simulink model "saturateModel_15b"  (R2015b)
settings: Solver=FixedStepAuto  SolverMode=SingleTasking  StartTime=0.0  StopTime=30.0  FixedStep=0.01  RelTol=1e-3
InitFcn:
  | init
StopFcn:
  | res_plot
values from neighbouring files (symbols this model uses):
  g = 9.8    [init.m]    (also in main.m)
  I_1 = 1.25    [init.m]
  I_2 = 1.25    [init.m]
  I_3 = 2.5    [init.m]
  k_1_phi = 5.5    [init.m]
  k_1_psi = 8.5    [init.m]
  k_1_theta = 5.5    [init.m]
  k_2_phi = 10    [init.m]
  k_2_psi = 20    [init.m]
  k_2_theta = 10    [init.m]
  K_4 = 0.012    [init.m]
  K_5 = 0.012    [init.m]
  K_6 = 0.012    [init.m]
  k_d_x = 2.5    [init.m]
  k_d_y = 2.5    [init.m]
  k_d_z = 4.5    [init.m]
  k_p_x = 1.8    [init.m]
  k_p_y = 1.8    [init.m]
  k_p_z = 5.5    [init.m]
  k_phi = 1    [init.m]
  k_psi = 1    [init.m]
  k_theta = 1    [init.m]
  l = 0.20    (= 0.2)    [init.m]
  m = 2    [init.m]    (also in main.m = 0.5)
  M_phi = 25    [init.m]
  M_psi = 25    [init.m]
  M_theta = 25    [init.m]
  state0 = [0;0;0;0;0;0;0;0;0;0;0;0]    [init.m]    (also in main.m = [0;0;0;0;0;0;0;0;0.1;0;0;0])
  state_des = [4;4;5;pi/4]    [init.m]
undefined symbols (not defined in the file or in its folder): c, kf
settings Model: Creator=KingBoy  LastModifiedBy=KingBoy
settings DataIOCC: LimitDataPoints=off
settings DebuggingCC: AllowSymbolicDim=on  SFUnexpectedBacktrackingDiag=error  SFNoUnconditionalDefaultTransitionDiag=error
settings ModelReferenceCC: PropagateSignalLabelsOutOfModel=on
settings GRTTargetCC: TargetLangStandard=C99 (ISO)
settings ConfigComp: CovMetricSettings=dwe  CovHtmlReporting=off  CovSaveCumulativeToWorkspaceVar=off  CovSaveSingleToWorkspaceVar=off  CovModelRefEnable=Off  CovExternalEMLEnable=on

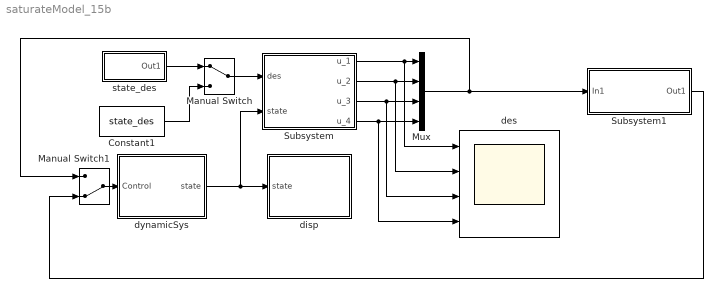
== system saturateModel_15b ==
  Constant1 : Constant  Value=state_des
  Manual Switch : ManualSwitch
  Manual Switch1 : ManualSwitch  CurrentSetting=0
  Mux : Mux
  Subsystem : Subsystem
  Subsystem1 : Subsystem
  des : Scope  NumInputPorts=4
  disp : Subsystem
  dynamicSys : Subsystem
  state_des : Subsystem
  wires:
  dynamicSys/1(state) -> disp/1(state), Subsystem/2(state)
  Constant1/1 -> Manual Switch/2
  Subsystem/1(u_1) -> des/1, Mux/1
  Subsystem/2(u_2) -> des/2, Mux/2
  Subsystem/3(u_3) -> des/3, Mux/3
  Subsystem/4(u_4) -> Mux/4, des/4
  Mux/1 -> Manual Switch1/1, Subsystem1/1(In1)
  state_des/1(Out1) -> Manual Switch/1
  Manual Switch/1 -> Subsystem/1(des)
  Subsystem1/1(Out1) -> Manual Switch1/2
  Manual Switch1/1 -> dynamicSys/1(Control)

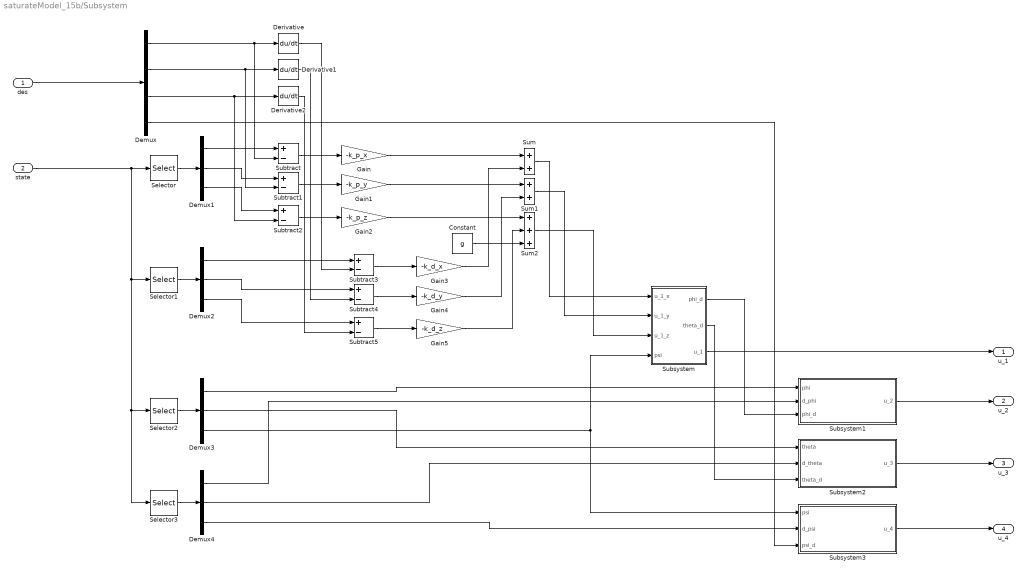
== system saturateModel_15b/Subsystem ==
  des : Inport
  state : Inport  Port=2
  Constant : Constant  Value=g
  Demux : Demux
  Demux{1..4} (4 alike) : Demux  Outputs=3
  Derivative : Derivative
  Derivative1 : Derivative
  Derivative2 : Derivative
  Gain : Gain  Gain=-k_p_x
  Gain1 : Gain  Gain=-k_p_y
  Gain2 : Gain  Gain=-k_p_z
  Gain3 : Gain  Gain=-k_d_x
  Gain4 : Gain  Gain=-k_d_y
  Gain5 : Gain  Gain=-k_d_z
  Selector : Selector  InputPortWidth=12  IndexOptions=Index vector (dialog)  Indices=[1:3]  OutputSizes=1
  Selector1 : Selector  InputPortWidth=12  IndexOptions=Index vector (dialog)  Indices=[4:6]  OutputSizes=1
  Selector2 : Selector  InputPortWidth=12  IndexOptions=Index vector (dialog)  Indices=[7:9]  OutputSizes=1
  Selector3 : Selector  InputPortWidth=12  IndexOptions=Index vector (dialog)  Indices=[10:12]  OutputSizes=1
  Subsystem : Subsystem
  Subsystem1 : Subsystem
  Subsystem2 : Subsystem
  Subsystem3 : Subsystem
  Subtract{,1..5} (6 alike) : Sum  Inputs=+-
  Sum : Sum
  Sum1 : Sum
  Sum2 : Sum  Inputs=+++
  u_1 : Outport
  u_2 : Outport  Port=2
  u_3 : Outport  Port=3
  u_4 : Outport  Port=4
  wires:
  state/1 -> Selector2/1, Selector3/1, Selector1/1, Selector/1
  des/1 -> Demux/1
  Demux/1 -> Subtract/2, Derivative/1
  Demux/2 -> Subtract1/2, Derivative1/1
  Demux/3 -> Subtract2/2, Derivative2/1
  Demux/4 -> Subsystem3/3(psi_d)
  Selector/1 -> Demux1/1
  Demux1/1 -> Subtract/1
  Demux1/2 -> Subtract1/1
  Demux1/3 -> Subtract2/1
  Selector1/1 -> Demux2/1
  Demux2/1 -> Subtract3/1
  Demux2/2 -> Subtract4/1
  Demux2/3 -> Subtract5/1
  Derivative/1 -> Subtract3/2
  Derivative1/1 -> Subtract4/2
  Derivative2/1 -> Subtract5/2
  Subtract/1 -> Gain/1
  Subtract2/1 -> Gain2/1
  Subtract1/1 -> Gain1/1
  Subtract3/1 -> Gain3/1
  Subtract4/1 -> Gain4/1
  Subtract5/1 -> Gain5/1
  Gain/1 -> Sum/1
  Gain1/1 -> Sum1/1
  Gain2/1 -> Sum2/1
  Gain3/1 -> Sum/2
  Gain4/1 -> Sum1/2
  Gain5/1 -> Sum2/2
  Constant/1 -> Sum2/3
  Selector2/1 -> Demux3/1
  Sum1/1 -> Subsystem/2(u_1_y)
  Sum/1 -> Subsystem/1(u_1_x)
  Demux3/3 -> Subsystem3/1(psi), Subsystem/4(psi)
  Sum2/1 -> Subsystem/3(u_1_z)
  Subsystem/3(u_1) -> u_1/1
  Subsystem/1(phi_d) -> Subsystem1/3(phi_d)
  Selector3/1 -> Demux4/1
  Demux4/1 -> Subsystem1/2(d_phi)
  Demux3/1 -> Subsystem1/1(phi)
  Demux3/2 -> Subsystem2/1(theta)
  Subsystem/2(theta_d) -> Subsystem2/3(theta_d)
  Demux4/2 -> Subsystem2/2(d_theta)
  Demux4/3 -> Subsystem3/2(d_psi)
  Subsystem3/1(u_4) -> u_4/1
  Subsystem1/1(u_2) -> u_2/1
  Subsystem2/1(u_3) -> u_3/1

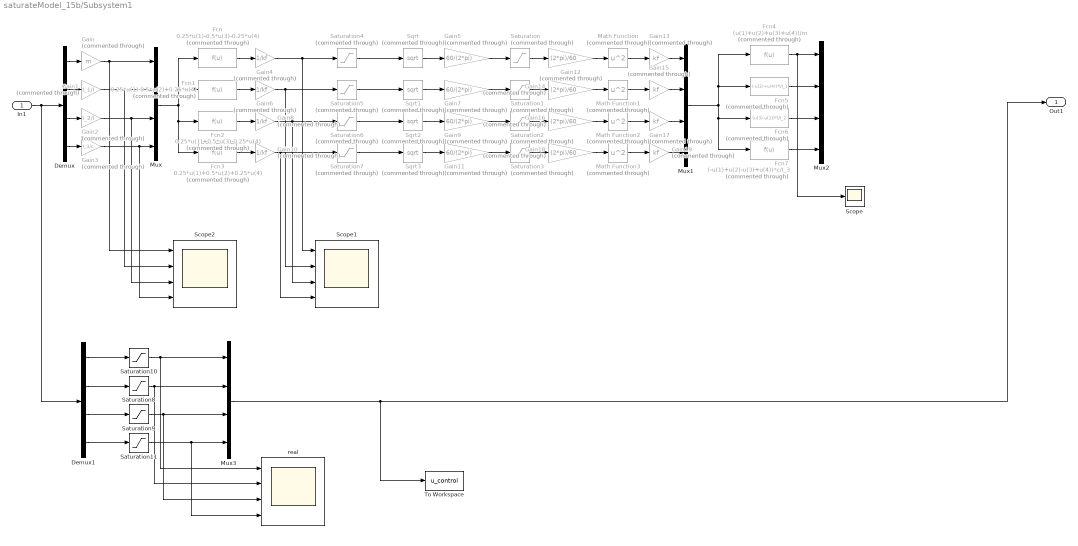
== system saturateModel_15b/Subsystem1 ==
  In1 : Inport
  Demux : Demux
  Demux1 : Demux
  Fcn : Fcn  Commented=through  Expr=0.25*u(1)-0.5*u(3)-0.25*u(4)
  Fcn1 : Fcn  Commented=through  Expr=0.25*u(1)-0.5*u(2)+0.25*u(4)
  Fcn2 : Fcn  Commented=through  Expr=0.25*u(1)+0.5*u(3)-0.25*u(4)
  Fcn3 : Fcn  Commented=through  Expr=0.25*u(1)+0.5*u(2)+0.25*u(4)
  Fcn4 : Fcn  Commented=through  Expr=(u(1)+u(2)+u(3)+u(4))/m
  Fcn5 : Fcn  Commented=through  Expr=(-u(2)+u(4))*l/I_1
  Fcn6 : Fcn  Commented=through  Expr=(u(3)-u(1))*l/I_2
  Fcn7 : Fcn  Commented=through  Expr=(-u(1)+u(2)-u(3)+u(4))*c/I_3
  Gain : Gain  Commented=through  Gain=m
  Gain1 : Gain  Commented=through  Gain=I_1/l
  Gain{4,6,8,10} (4 alike) : Gain  Commented=through  Gain=1/kf
  Gain{5,7,9,11} (4 alike) : Gain  Commented=through  Gain=60/(2*pi)
  Gain{12,14,16,18} (4 alike) : Gain  Commented=through  Gain=(2*pi)/60
  Gain{13,15,17,19} (4 alike) : Gain  Commented=through  Gain=kf
  Gain2 : Gain  Commented=through  Gain=I_2/l
  Gain3 : Gain  Commented=through  Gain=I_3/c
  Math Function{,1..3} (4 alike) : Math  Commented=through  Operator=square  SaturateOnIntegerOverflow=on
  Mux{,1..3} (4 alike) : Mux
  Saturation{,1..3} (4 alike) : Saturate  Commented=through  UpperLimit=24000  LowerLimit=0
  Saturation10 : Saturate  UpperLimit=2e-3*4*(20000*2*pi/60)^2/2  LowerLimit=0
  Saturation11 : Saturate  UpperLimit=4*1e-3*(20000*2*pi/60)^2/2.5  LowerLimit=-4*1e-3*(20000*2*pi/60)^2/2.5
  Saturation{4..7} (4 alike) : Saturate  Commented=through  UpperLimit=inf  LowerLimit=0
  Saturation8 : Saturate  UpperLimit=2e-3*0.2*(20000*2*pi/60)^2/1.25  LowerLimit=-2e-3*0.2*(20000*2*pi/60)^2/1.25
  Saturation9 : Saturate  UpperLimit=2e-3*0.2*(20000*2*pi/60)^2/1.25  LowerLimit=-2e-3*0.2*(20000*2*pi/60)^2/1.25
  Scope : Scope
  Scope1 : Scope  NumInputPorts=4
  Scope2 : Scope  NumInputPorts=4
  Sqrt{,1..3} (4 alike) : Sqrt  Commented=through  SaturateOnIntegerOverflow=on
  To Workspace : ToWorkspace  VariableName=u_control  SampleTime=-1
  real : Scope  NumInputPorts=4
  Out1 : Outport
  wires:
  In1/1 -> Demux1/1, Demux/1
  Demux/1 -> Gain/1
  Demux/2 -> Gain1/1
  Demux/3 -> Gain2/1
  Demux/4 -> Gain3/1
  Gain1/1 -> Mux/2, Scope2/2
  Gain2/1 -> Mux/3, Scope2/3
  Mux/1 -> Fcn3/1, Fcn2/1, Fcn1/1, Fcn/1
  Fcn/1 -> Gain4/1
  Gain4/1 -> Scope1/1, Saturation4/1
  Sqrt/1 -> Gain5/1
  Gain5/1 -> Saturation/1
  Gain7/1 -> Saturation1/1
  Sqrt1/1 -> Gain7/1
  Gain6/1 -> Scope1/2, Saturation5/1
  Fcn1/1 -> Gain6/1
  Gain8/1 -> Scope1/3, Saturation6/1
  Sqrt2/1 -> Gain9/1
  Gain9/1 -> Saturation2/1
  Gain11/1 -> Saturation3/1
  Sqrt3/1 -> Gain11/1
  Gain10/1 -> Scope1/4, Saturation7/1
  Fcn3/1 -> Gain10/1
  Fcn2/1 -> Gain8/1
  Saturation/1 -> Gain12/1
  Gain12/1 -> Math Function/1
  Math Function/1 -> Gain13/1
  Math Function1/1 -> Gain15/1
  Gain14/1 -> Math Function1/1
  Saturation1/1 -> Gain14/1
  Gain16/1 -> Math Function2/1
  Math Function2/1 -> Gain17/1
  Saturation2/1 -> Gain16/1
  Math Function3/1 -> Gain19/1
  Gain18/1 -> Math Function3/1
  Saturation3/1 -> Gain18/1
  Gain13/1 -> Mux1/1
  Gain15/1 -> Mux1/2
  Gain17/1 -> Mux1/3
  Gain19/1 -> Mux1/4
  Mux1/1 -> Fcn7/1, Fcn6/1, Fcn5/1, Fcn4/1
  Fcn6/1 -> Mux2/3
  Fcn7/1 -> Mux2/4
  Fcn5/1 -> Mux2/2
  Fcn4/1 -> Mux2/1, Scope/1
  Gain/1 -> Mux/1, Scope2/1
  Gain3/1 -> Mux/4, Scope2/4
  Saturation4/1 -> Sqrt/1
  Saturation5/1 -> Sqrt1/1
  Saturation6/1 -> Sqrt2/1
  Saturation7/1 -> Sqrt3/1
  Demux1/2 -> Saturation8/1
  Demux1/3 -> Saturation9/1
  Demux1/1 -> Saturation10/1
  Saturation10/1 -> real/1, Mux3/1
  Saturation8/1 -> real/2, Mux3/2
  Saturation9/1 -> real/3, Mux3/3
  Demux1/4 -> Saturation11/1
  Mux3/1 -> To Workspace/1, Out1/1
  Saturation11/1 -> real/4, Mux3/4

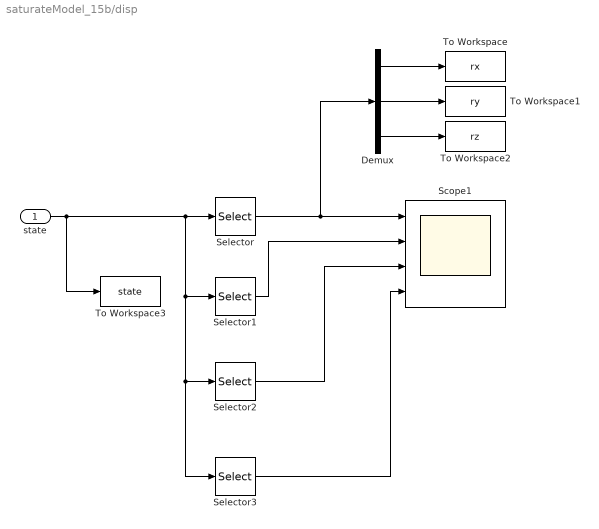
== system saturateModel_15b/disp ==
  state : Inport
  Demux : Demux  Outputs=3
  Scope1 : Scope  NumInputPorts=4
  Selector : Selector  InputPortWidth=12  IndexOptions=Index vector (dialog)  Indices=[1:3]  OutputSizes=1
  Selector1 : Selector  InputPortWidth=12  IndexOptions=Index vector (dialog)  Indices=[4:6]  OutputSizes=1
  Selector2 : Selector  InputPortWidth=12  IndexOptions=Index vector (dialog)  Indices=[7:9]  OutputSizes=1
  Selector3 : Selector  InputPortWidth=12  IndexOptions=Index vector (dialog)  Indices=[10:12]  OutputSizes=1
  To Workspace : ToWorkspace  VariableName=rx  SampleTime=-1
  To Workspace1 : ToWorkspace  VariableName=ry  SampleTime=-1
  To Workspace2 : ToWorkspace  VariableName=rz  SampleTime=-1
  To Workspace3 : ToWorkspace  VariableName=state  SampleTime=-1
  wires:
  Selector3/1 -> Scope1/4
  Selector/1 -> Demux/1, Scope1/1
  Selector1/1 -> Scope1/2
  Selector2/1 -> Scope1/3
  state/1 -> To Workspace3/1, Selector2/1, Selector3/1, Selector1/1, Selector/1
  Demux/1 -> To Workspace/1
  Demux/2 -> To Workspace1/1
  Demux/3 -> To Workspace2/1

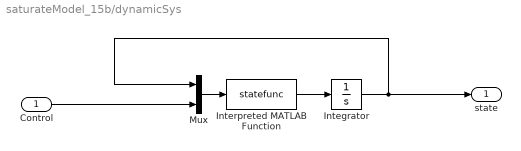
== system saturateModel_15b/dynamicSys ==
  Control : Inport
  Integrator : Integrator  InitialCondition=state0
  Interpreted MATLAB Function : MATLABFcn  MATLABFcn=statefunc  OutputDimensions=12
  Mux : Mux  Inputs=2
  state : Outport
  wires:
  Mux/1 -> Interpreted MATLAB Function/1
  Integrator/1 -> state/1, Mux/1
  Interpreted MATLAB Function/1 -> Integrator/1
  Control/1 -> Mux/2

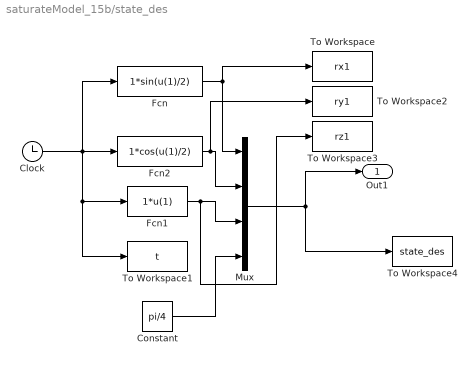
== system saturateModel_15b/state_des ==
  Clock : Clock
  Constant : Constant  Value=pi/4
  Fcn : Fcn  Expr=1*sin(u(1)/2)
  Fcn1 : Fcn  Expr=1*u(1)
  Fcn2 : Fcn  Expr=1*cos(u(1)/2)
  Mux : Mux
  To Workspace : ToWorkspace  VariableName=rx1  SampleTime=-1
  To Workspace1 : ToWorkspace  VariableName=t  SampleTime=-1
      settings: Save2DSignal=2-D array (concatenate along first dimension)
  To Workspace2 : ToWorkspace  VariableName=ry1  SampleTime=-1
  To Workspace3 : ToWorkspace  VariableName=rz1  SampleTime=-1
  To Workspace4 : ToWorkspace  VariableName=state_des  SampleTime=-1
  Out1 : Outport
  wires:
  Mux/1 -> To Workspace4/1, Out1/1
  Fcn2/1 -> To Workspace2/1, Mux/2
  Fcn1/1 -> To Workspace3/1, Mux/3
  Clock/1 -> To Workspace1/1, Fcn1/1, Fcn/1, Fcn2/1
  Fcn/1 -> To Workspace/1, Mux/1
  Constant/1 -> Mux/4

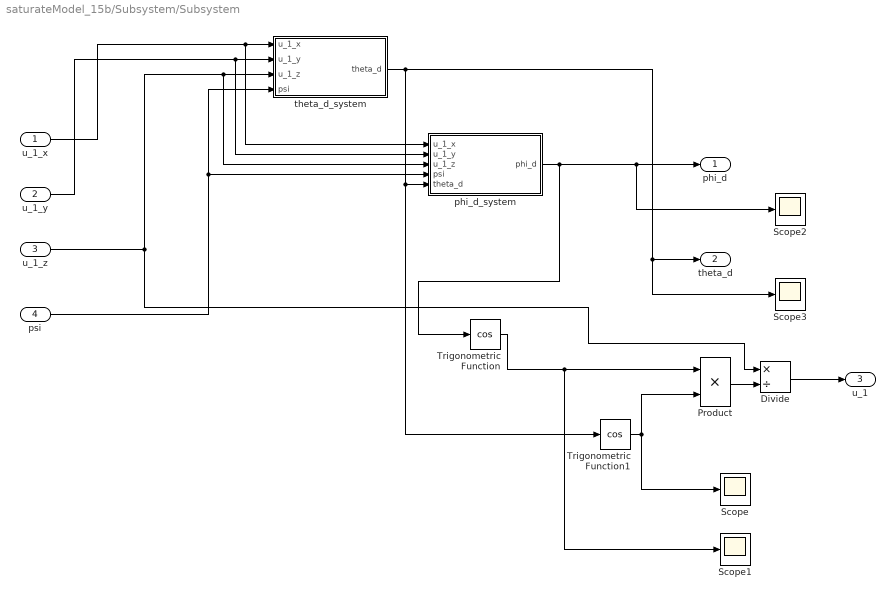
== system saturateModel_15b/Subsystem/Subsystem ==
  u_1_x : Inport
  u_1_y : Inport  Port=2
  u_1_z : Inport  Port=3
  psi : Inport  Port=4
  Divide : Product  Inputs=*/
  Product : Product
  Scope{,1..3} (4 alike) : Scope
  Trigonometric Function : Trigonometry  Operator=cos
  Trigonometric Function1 : Trigonometry  Operator=cos
  phi_d_system : Subsystem
  theta_d_system : Subsystem
  phi_d : Outport
  theta_d : Outport  Port=2
  u_1 : Outport  Port=3
  wires:
  Product/1 -> Divide/2
  u_1_x/1 -> theta_d_system/1(u_1_x), phi_d_system/1(u_1_x)
  u_1_y/1 -> theta_d_system/2(u_1_y), phi_d_system/2(u_1_y)
  u_1_z/1 -> Divide/1, phi_d_system/3(u_1_z), theta_d_system/3(u_1_z)
  psi/1 -> phi_d_system/4(psi), theta_d_system/4(psi)
  phi_d_system/1(phi_d) -> Trigonometric Function/1, Scope2/1, phi_d/1
  theta_d_system/1(theta_d) -> Trigonometric Function1/1, phi_d_system/5(theta_d), Scope3/1, theta_d/1
  Trigonometric Function/1 -> Scope1/1, Product/1
  Trigonometric Function1/1 -> Scope/1, Product/2
  Divide/1 -> u_1/1

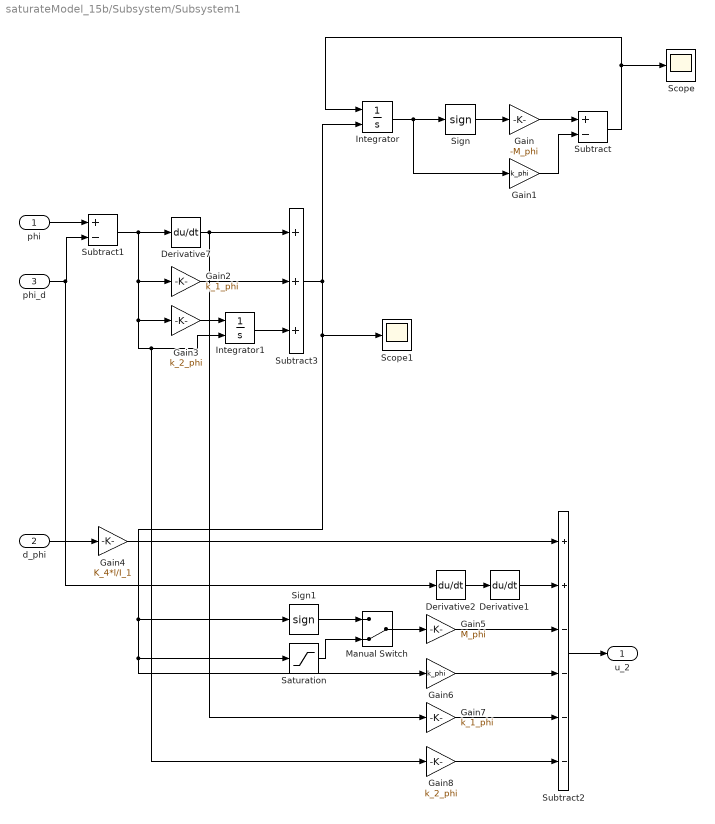
== system saturateModel_15b/Subsystem/Subsystem1 ==
  phi : Inport
  d_phi : Inport  Port=2
  phi_d : Inport  Port=3
  Derivative1 : Derivative
  Derivative2 : Derivative
  Derivative7 : Derivative
  Gain : Gain  Gain=-M_phi
  Gain1 : Gain  Gain=k_phi
  Gain2 : Gain  Gain=k_1_phi
  Gain3 : Gain  Gain=k_2_phi
  Gain4 : Gain  Gain=K_4*l/I_1
  Gain5 : Gain  Gain=M_phi
  Gain6 : Gain  Gain=k_phi
  Gain7 : Gain  Gain=k_1_phi
  Gain8 : Gain  Gain=k_2_phi
  Integrator : Integrator  InitialConditionSource=external
  Integrator1 : Integrator  InitialConditionSource=external
  Manual Switch : ManualSwitch  CurrentSetting=0
  Saturation : Saturate  UpperLimit=1  LowerLimit=-1
  Scope : Scope
  Scope1 : Scope
  Sign : Signum  ZeroCross=off
  Sign1 : Signum  ZeroCross=off
  Subtract : Sum  Inputs=+-
  Subtract1 : Sum  Inputs=+-
  Subtract2 : Sum  Inputs=++----
  Subtract3 : Sum  Inputs=+++
  u_2 : Outport
  wires:
  Gain1/1 -> Subtract/2
  Integrator/1 -> Gain1/1, Sign/1
  Subtract/1 -> Scope/1, Integrator/1
  Gain/1 -> Subtract/1
  Sign/1 -> Gain/1
  phi/1 -> Subtract1/1
  phi_d/1 -> Derivative2/1, Subtract1/2
  Subtract1/1 -> Gain3/1, Gain8/1, Integrator1/2, Gain2/1, Derivative7/1
  Derivative7/1 -> Gain7/1, Subtract3/1
  Gain2/1 -> Subtract3/2
  Integrator1/1 -> Subtract3/3
  Gain3/1 -> Integrator1/1
  Derivative1/1 -> Subtract2/2
  d_phi/1 -> Gain4/1
  Gain4/1 -> Subtract2/1
  Derivative2/1 -> Derivative1/1
  Gain5/1 -> Subtract2/3
  Gain6/1 -> Subtract2/4
  Subtract3/1 -> Sign1/1, Saturation/1, Gain6/1, Scope1/1, Integrator/2
  Gain8/1 -> Subtract2/6
  Gain7/1 -> Subtract2/5
  Subtract2/1 -> u_2/1
  Saturation/1 -> Manual Switch/2
  Sign1/1 -> Manual Switch/1
  Manual Switch/1 -> Gain5/1

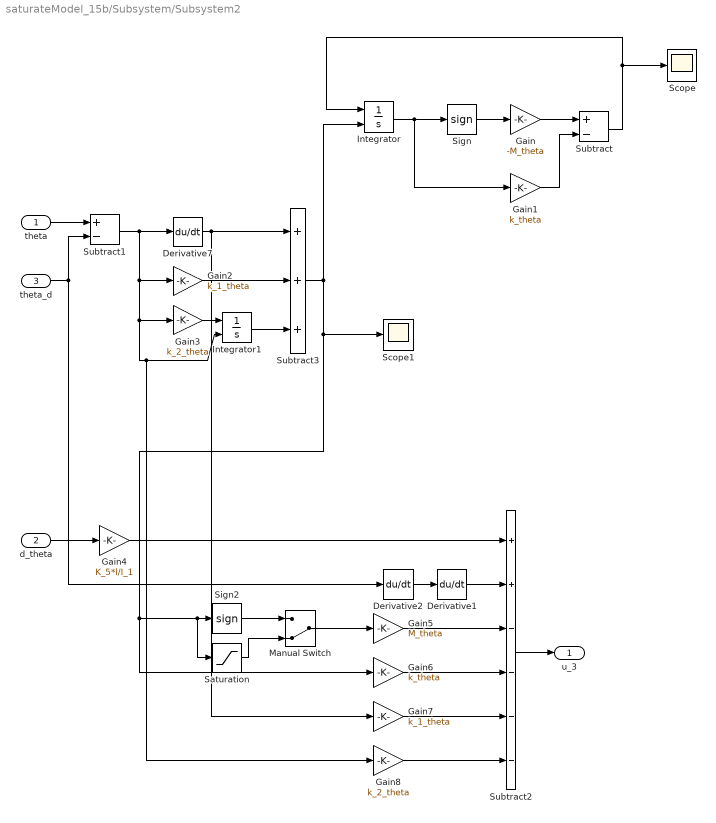
== system saturateModel_15b/Subsystem/Subsystem2 ==
  theta : Inport
  d_theta : Inport  Port=2
  theta_d : Inport  Port=3
  Derivative1 : Derivative
  Derivative2 : Derivative
  Derivative7 : Derivative
  Gain : Gain  Gain=-M_theta
  Gain1 : Gain  Gain=k_theta
  Gain2 : Gain  Gain=k_1_theta
  Gain3 : Gain  Gain=k_2_theta
  Gain4 : Gain  Gain=K_5*l/I_1
  Gain5 : Gain  Gain=M_theta
  Gain6 : Gain  Gain=k_theta
  Gain7 : Gain  Gain=k_1_theta
  Gain8 : Gain  Gain=k_2_theta
  Integrator : Integrator  InitialConditionSource=external
  Integrator1 : Integrator  InitialConditionSource=external
  Manual Switch : ManualSwitch  CurrentSetting=0
  Saturation : Saturate  UpperLimit=1  LowerLimit=-1
  Scope : Scope
  Scope1 : Scope
  Sign : Signum  ZeroCross=off
  Sign2 : Signum  ZeroCross=off
  Subtract : Sum  Inputs=+-
  Subtract1 : Sum  Inputs=+-
  Subtract2 : Sum  Inputs=++----
  Subtract3 : Sum  Inputs=+++
  u_3 : Outport
  wires:
  Integrator1/1 -> Subtract3/3
  Gain2/1 -> Subtract3/2
  theta/1 -> Subtract1/1
  Sign/1 -> Gain/1
  Gain/1 -> Subtract/1
  Subtract/1 -> Integrator/1, Scope/1
  Integrator/1 -> Sign/1, Gain1/1
  Gain1/1 -> Subtract/2
  Gain3/1 -> Integrator1/1
  Gain7/1 -> Subtract2/5
  Manual Switch/1 -> Gain5/1
  Derivative7/1 -> Gain7/1, Subtract3/1
  Subtract2/1 -> u_3/1
  Subtract3/1 -> Integrator/2, Gain6/1, Saturation/1, Sign2/1, Scope1/1
  Gain4/1 -> Subtract2/1
  d_theta/1 -> Gain4/1
  theta_d/1 -> Derivative2/1, Subtract1/2
  Gain6/1 -> Subtract2/4
  Gain5/1 -> Subtract2/3
  Subtract1/1 -> Derivative7/1, Gain2/1, Gain8/1, Integrator1/2, Gain3/1
  Derivative2/1 -> Derivative1/1
  Gain8/1 -> Subtract2/6
  Derivative1/1 -> Subtract2/2
  Saturation/1 -> Manual Switch/2
  Sign2/1 -> Manual Switch/1

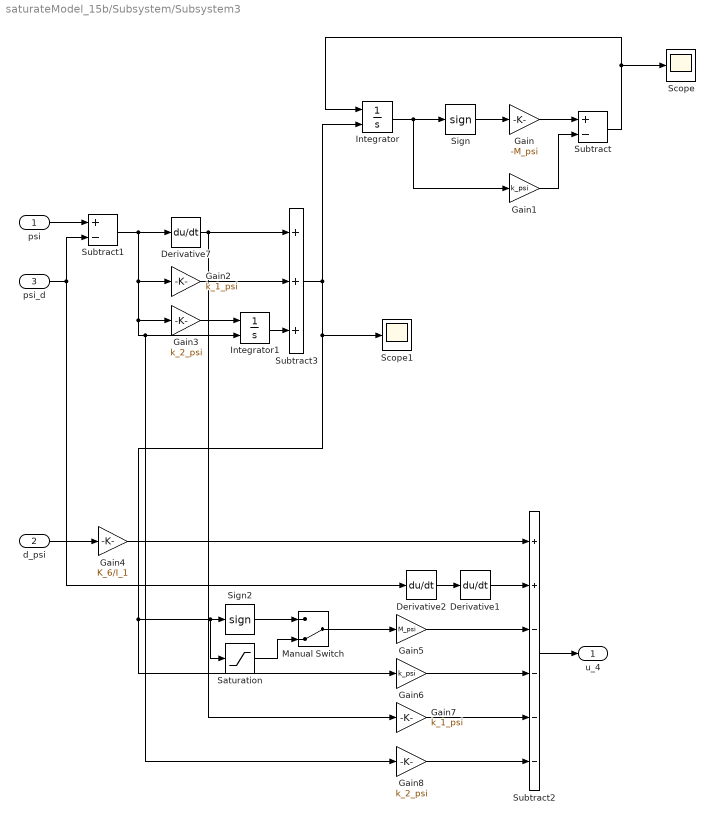
== system saturateModel_15b/Subsystem/Subsystem3 ==
  psi : Inport
  d_psi : Inport  Port=2
  psi_d : Inport  Port=3
  Derivative1 : Derivative
  Derivative2 : Derivative
  Derivative7 : Derivative
  Gain : Gain  Gain=-M_psi
  Gain1 : Gain  Gain=k_psi
  Gain2 : Gain  Gain=k_1_psi
  Gain3 : Gain  Gain=k_2_psi
  Gain4 : Gain  Gain=K_6/I_1
  Gain5 : Gain  Gain=M_psi
  Gain6 : Gain  Gain=k_psi
  Gain7 : Gain  Gain=k_1_psi
  Gain8 : Gain  Gain=k_2_psi
  Integrator : Integrator  InitialConditionSource=external
  Integrator1 : Integrator  InitialConditionSource=external
  Manual Switch : ManualSwitch  CurrentSetting=0
  Saturation : Saturate  UpperLimit=1  LowerLimit=-1
  Scope : Scope
  Scope1 : Scope
  Sign : Signum  ZeroCross=off
  Sign2 : Signum  ZeroCross=off
  Subtract : Sum  Inputs=+-
  Subtract1 : Sum  Inputs=+-
  Subtract2 : Sum  Inputs=++----
  Subtract3 : Sum  Inputs=+++
  u_4 : Outport
  wires:
  Gain1/1 -> Subtract/2
  Integrator/1 -> Gain1/1, Sign/1
  Subtract/1 -> Scope/1, Integrator/1
  Gain/1 -> Subtract/1
  Sign/1 -> Gain/1
  psi/1 -> Subtract1/1
  Gain2/1 -> Subtract3/2
  Integrator1/1 -> Subtract3/3
  Gain3/1 -> Integrator1/1
  Derivative7/1 -> Gain7/1, Subtract3/1
  Derivative1/1 -> Subtract2/2
  Gain8/1 -> Subtract2/6
  Gain6/1 -> Subtract2/4
  Gain5/1 -> Subtract2/3
  Gain7/1 -> Subtract2/5
  Derivative2/1 -> Derivative1/1
  Subtract2/1 -> u_4/1
  Gain4/1 -> Subtract2/1
  Subtract3/1 -> Gain6/1, Saturation/1, Sign2/1, Scope1/1, Integrator/2
  d_psi/1 -> Gain4/1
  psi_d/1 -> Derivative2/1, Subtract1/2
  Subtract1/1 -> Gain3/1, Gain8/1, Integrator1/2, Gain2/1, Derivative7/1
  Manual Switch/1 -> Gain5/1
  Sign2/1 -> Manual Switch/1
  Saturation/1 -> Manual Switch/2

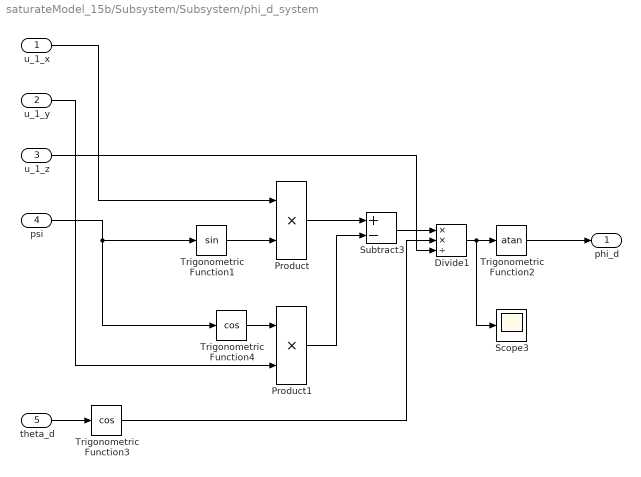
== system saturateModel_15b/Subsystem/Subsystem/phi_d_system ==
  u_1_x : Inport
  u_1_y : Inport  Port=2
  u_1_z : Inport  Port=3
  psi : Inport  Port=4
  theta_d : Inport  Port=5
  Divide1 : Product  Inputs=**/
  Product : Product
  Product1 : Product
  Scope3 : Scope
  Subtract3 : Sum  Inputs=+-
  Trigonometric Function1 : Trigonometry
  Trigonometric Function2 : Trigonometry  Operator=atan
  Trigonometric Function3 : Trigonometry  Operator=cos
  Trigonometric Function4 : Trigonometry  Operator=cos
  phi_d : Outport
  wires:
  Product/1 -> Subtract3/1
  u_1_x/1 -> Product/1
  psi/1 -> Trigonometric Function4/1, Trigonometric Function1/1
  Trigonometric Function1/1 -> Product/2
  Divide1/1 -> Scope3/1, Trigonometric Function2/1
  Trigonometric Function2/1 -> phi_d/1
  Subtract3/1 -> Divide1/1
  u_1_y/1 -> Product1/2
  u_1_z/1 -> Divide1/3
  Product1/1 -> Subtract3/2
  theta_d/1 -> Trigonometric Function3/1
  Trigonometric Function4/1 -> Product1/1
  Trigonometric Function3/1 -> Divide1/2

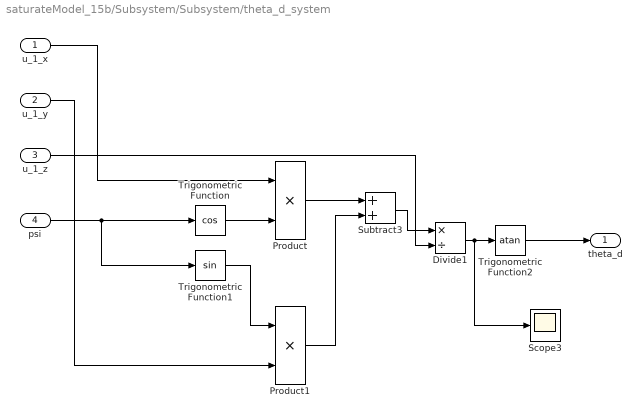
== system saturateModel_15b/Subsystem/Subsystem/theta_d_system ==
  u_1_x : Inport
  u_1_y : Inport  Port=2
  u_1_z : Inport  Port=3
  psi : Inport  Port=4
  Divide1 : Product  Inputs=*/
  Product : Product
  Product1 : Product
  Scope3 : Scope
  Subtract3 : Sum
  Trigonometric Function : Trigonometry  Operator=cos
  Trigonometric Function1 : Trigonometry
  Trigonometric Function2 : Trigonometry  Operator=atan
  theta_d : Outport
  wires:
  Product1/1 -> Subtract3/2
  Trigonometric Function/1 -> Product/2
  u_1_z/1 -> Divide1/2
  Subtract3/1 -> Divide1/1
  Trigonometric Function2/1 -> theta_d/1
  Divide1/1 -> Scope3/1, Trigonometric Function2/1
  psi/1 -> Trigonometric Function/1, Trigonometric Function1/1
  u_1_x/1 -> Product/1
  Product/1 -> Subtract3/1
  Trigonometric Function1/1 -> Product1/1
  u_1_y/1 -> Product1/2
